simulink model "example_DataFromFile_inSubsystem"  (R2018b)
settings: Solver=ode45  StartTime=0.0  StopTime=24*3600  RelTol=1e-3  EnableMultiTasking=on
undefined symbols (not defined in the file): path_carnot
libraries: carnot x2
settings Model: Creator=drhf  LastModifiedBy=drhf
settings DataIOCC: LimitDataPoints=on  SaveFormat=Array
settings OptimizationCC: ExpressionDepthLimit=2147483647  LifeSpan=inf
settings DebuggingCC: UnderspecifiedInitializationDetection=Classic  MergeDetectMultiDrivingBlocksExec=none  StateNameClashWarn=warning  SFUnexpectedBacktrackingDiag=warning  SFNoUnconditionalDefaultTransitionDiag=warning  SFExecutionAtInitializationDiag=none
settings HardwareCC: ProdBitPerPointer=32  ProdBitPerSizeT=32  ProdBitPerPtrDiffT=32  ProdLargestAtomicFloat=None  ProdIntDivRoundTo=Undefined  ProdEndianess=Unspecified  ProdWordSize=32  ProdHWDeviceType=32-bit Generic
settings ModelReferenceCC: PropagateSignalLabelsOutOfModel=off
settings SFSimCC: SimUseLocalCustomCode=off
settings RTWCC: RTWUseLocalCustomCode=off
settings CodeAppCC: StateflowObjectComments=on
settings GRTTargetCC: TargetLangStandard=C89/C90 (ANSI)  GeneratePreprocessorConditionals=Disable all  CombineOutputUpdateFcns=off  GRTInterface=on
settings ConfigComp: CovMetricSettings=dw  CovHtmlReporting=on  CovSaveCumulativeToWorkspaceVar=on  CovSaveSingleToWorkspaceVar=on  CovExternalEMLEnable=off

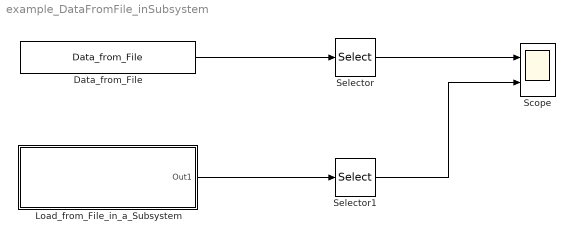
== system example_DataFromFile_inSubsystem ==
  Data_from_File : carnot/Load/General/Data_from_File  PathName=path_carnot('data')  FileName='DE_TRY2010_06_averageYear.mat'  UserParam=off  DataName=DataName  t_sample=60
      settings: SourceProductName=Carnot
  Load_from_File_in_a_Subsystem : Subsystem  mask{PathName=path_carnot('data'), FileName='DE_TRY2010_06_averageYear.mat'}
      mask prompts: PathName "Selected path"; FileName "File"
      mask TypeOptions PathName: Data_from_File1/PathName
      mask TypeOptions FileName: Data_from_File1/FileName
  Scope : Scope  NumInputPorts=2
  Selector : Selector  InputPortWidth=18  IndexOptions=Index vector (dialog)  Indices=[7]  OutputSizes=1
  Selector1 : Selector  InputPortWidth=18  IndexOptions=Index vector (dialog)  Indices=[7]  OutputSizes=1
  wires:
  Data_from_File/1 -> Selector/1
  Selector/1 -> Scope/1
  Selector1/1 -> Scope/2
  Load_from_File_in_a_Subsystem/1(Out1) -> Selector1/1

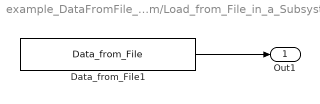
== system example_DataFromFile_inSubsystem/Load_from_File_in_a_Subsystem ==
  Data_from_File1 : carnot/Load/General/Data_from_File  PathName=PathName  FileName=FileName  UserParam=on  DataName=DataName  t_sample=60
      settings: SourceProductName=Carnot
  Out1 : Outport
  wires:
  Data_from_File1/1 -> Out1/1
